simulink model "PubIfChassisHMI_MDL_DS"  (R2020b)
settings: configuration reference "DspaceConfig" (kept outside this file)
PostLoadFcn:
  | if any(exist('dsrtsu_mdlpostloadfcn', 'file') ~= 0), dsrtsu_mdlpostloadfcn('Execute', bdroot); end
InitFcn:
  | , if any(exist('rtifpga_mdlclblib', 'file') ~= 0), rtifpga_mdlclblib('Init', bdroot); end,
  | , if any(exist('dsmpb_private', 'file') ~= 0), dsmpb_private('dsmpb_mdlclblib', 'Init', bdroot); end,
PreSaveFcn:
  | , if any(exist('dsmpb_private', 'file') ~= 0), dsmpb_private('dsmpb_mdlclblib', 'PreSave', bdroot); end,
CloseFcn:
  | , if any(exist('dsmpb_private', 'file') ~= 0), dsmpb_private('dsmpb_mdlclblib', 'Close', bdroot); end,
settings Model: DataDictionary=HMI_Parameter.sldd  RTICANMMDATA=struct('GeneralSetupData',struct('modelroot','E:\HWA_Project\Git_ADAS_Store\projcct\adas_project\AdasModel_DSconfig','generalsettings',struct('filesettings',struct('destfolder',struct('Name','RTICANMM_FILES','Check',1),'buildfolder',struct('Name','.','Check',1),'AbsDestfolder',struct('Name','E:\HWA_Project\Git_ADAS_Store\projcct\adas_project\AdasModel_DSconfig\RTICANMM_FILES'),'AbsBuildfolder',struct('Name','E:\HWA_Project\Git_ADAS_Store\projcct\adas_project\AdasModel_DSconfig'))),'options',struct('addpaths',1,'rmpaths',1,'addtrcexclusion',false,'cannavigator',struct('checkmonitoring',0),'show_usrtrc',0,'use_usrtrc',0),'advanced',struct('options',ones(1,100)),'MPSetup',{{}},'RTI',struct('Type','DSRT','Ver','4.4','Date','02-Nov-2020'),'modelname','PubIfChassisHMI_MDL_DS','block','PubIfChassisHMI_MDL_DS'))  DSRTSU_INTERNAL_RTIFPGA=170  Creator=GW00180895  LastModifiedBy=GW00201299
settings ConfigSetRef: SourceName=DspaceConfig

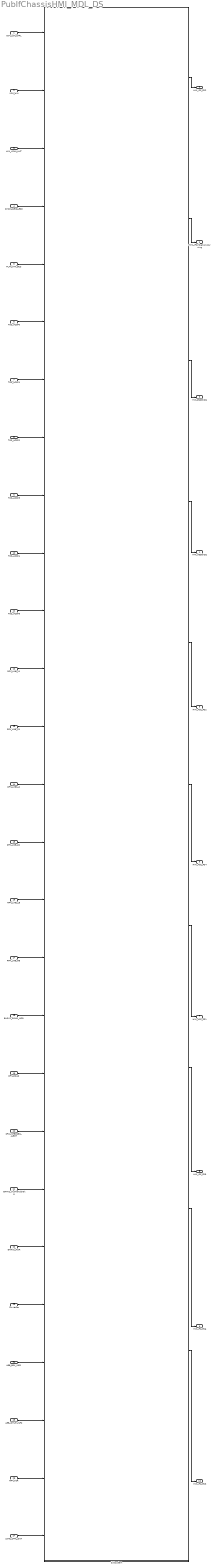
== system PubIfChassisHMI_MDL_DS ==
  VSM_LON_CTRL : Inport  OutDataTypeStr=Bus: VSM_LON_CTRL_BUS  PortDimensions=1  BusOutputAsStruct=on
  VSM_HMI : Inport  Port=2  OutDataTypeStr=Bus: VSM_HMI_BUS  PortDimensions=1  BusOutputAsStruct=on
  HMI_VCAN_HUT : Inport  Port=3  OutDataTypeStr=Bus: VCAN_HUT_MSG_BUS  PortDimensions=1  BusOutputAsStruct=on
  DMON_SENS_ERR : Inport  Port=4  OutDataTypeStr=Bus: DMON_SENS_ERR_BUS  PortDimensions=1  BusOutputAsStruct=on
  PLAN_HMI_BUS : Inport  Port=5  OutDataTypeStr=Bus: PLAN_HMI_BUS  PortDimensions=1  BusOutputAsStruct=on
  TOS_ACCP0 : Inport  Port=6  OutDataTypeStr=Bus: TOS_ACCP0_BUS  PortDimensions=1  BusOutputAsStruct=on
  TOS_ACCP1 : Inport  Port=7  OutDataTypeStr=Bus: TOS_ACCP1_BUS  PortDimensions=1  BusOutputAsStruct=on
  TOS_ACCP2 : Inport  Port=8  OutDataTypeStr=Bus: TOS_ACCP2_BUS  PortDimensions=1  BusOutputAsStruct=on
  TOS_ACCP3 : Inport  Port=9  OutDataTypeStr=Bus: TOS_ACCP3_BUS  PortDimensions=1  BusOutputAsStruct=on
  TOS_ACCP4 : Inport  Port=10  OutDataTypeStr=Bus: TOS_ACCP4_BUS  PortDimensions=1  BusOutputAsStruct=on
  TOS_ACCP5 : Inport  Port=11  OutDataTypeStr=Bus: TOS_ACCP5_BUS  PortDimensions=1  BusOutputAsStruct=on
  RFM_LINE_L1 : Inport  Port=12  OutDataTypeStr=Bus: RFM_LINE_BUS  PortDimensions=1  BusOutputAsStruct=on
  RFM_LINE_R1 : Inport  Port=13  OutDataTypeStr=Bus: RFM_LINE_BUS  PortDimensions=1  BusOutputAsStruct=on
  RFM_LINE_L2 : Inport  Port=14  OutDataTypeStr=Bus: RFM_LINE_BUS  PortDimensions=1  BusOutputAsStruct=on
  RFM_LINE_R2 : Inport  Port=15  OutDataTypeStr=Bus: RFM_LINE_BUS  PortDimensions=1  BusOutputAsStruct=on
  RFM_LINE_LB : Inport  Port=16  OutDataTypeStr=Bus: RFM_LINE_BUS  PortDimensions=1  BusOutputAsStruct=on
  RFM_LINE_RB : Inport  Port=17  OutDataTypeStr=Bus: RFM_LINE_BUS  PortDimensions=1  BusOutputAsStruct=on
  EHRV2_ROAD_INFO : Inport  Port=18  OutDataTypeStr=Bus: EHRV2_ROAD_INFO_BUS  PortDimensions=1  BusOutputAsStruct=on
  RFM_ROAD : Inport  Port=19  OutDataTypeStr=Bus: RFM_ROAD_BUS  PortDimensions=1  BusOutputAsStruct=on
  RFM_INTERSEC_ALERT : Inport  Port=20  OutDataTypeStr=Bus: RFM_INTERSEC_ALERT_BUS  PortDimensions=1  BusOutputAsStruct=on
  EHRV2_HutHandshake : Inport  Port=21  OutDataTypeStr=uint8  PortDimensions=1  BusOutputAsStruct=on
  EHRV2_HDR : Inport  Port=22  OutDataTypeStr=Bus: EHRV2_HDR_BUS  PortDimensions=1  BusOutputAsStruct=on
  DriverSts : Inport  Port=23  OutDataTypeStr=uint8  PortDimensions=1  BusOutputAsStruct=on
  AEB_BRK_INFO : Inport  Port=24  OutDataTypeStr=Bus: AEB_BRK_INFO_BUS  PortDimensions=1  BusOutputAsStruct=on
  AEB_IPHUT_INFO : Inport  Port=25  OutDataTypeStr=Bus: AEB_IPHUT_INFO_BUS  PortDimensions=1  BusOutputAsStruct=on
  RFM_TSR : Inport  Port=26  OutDataTypeStr=Bus: RFM_TSR_BUS  PortDimensions=1  BusOutputAsStruct=on
  LONC_CTRL_OUT : Inport  Port=27  OutDataTypeStr=Bus: LONC_CTRL_OUT_BUS  PortDimensions=1  BusOutputAsStruct=on
  Subsystem : Subsystem  ReferencedSubsystem=PvtSubSys_HMI
  HMI_IFC_FD2 : Outport  OutDataTypeStr=Bus: HMI_IFC_FD2_BUS  PortDimensions=1  BusOutputAsStruct=on
  HMI_IFCVibrationWarning : Outport  Port=2  OutDataTypeStr=uint8  PortDimensions=1  BusOutputAsStruct=on
  HMI_ESSErrSts : Outport  Port=3  OutDataTypeStr=boolean  BusOutputAsStruct=on
  HMI_AESErrSts : Outport  Port=4  OutDataTypeStr=boolean  BusOutputAsStruct=on
  HMI_ACC_FD2 : Outport  Port=5  OutDataTypeStr=Bus: HMI_ACC_FD2_BUS  PortDimensions=1  BusOutputAsStruct=on
  HMI_ACC_FD4 : Outport  Port=6  OutDataTypeStr=Bus: HMI_ACC_FD4_BUS  PortDimensions=1  BusOutputAsStruct=on
  HMI_ACC_FD1 : Outport  Port=7  OutDataTypeStr=Bus: HMI_ACC_FD1_BUS  PortDimensions=1  BusOutputAsStruct=on
  HMI_IFC_FD5 : Outport  Port=8  OutDataTypeStr=Bus: HMI_IFC_FD5_BUS  PortDimensions=1  BusOutputAsStruct=on
  HMI_IFC_FD6 : Outport  Port=9  OutDataTypeStr=Bus: HMI_IFC_FD6_BUS  PortDimensions=1  BusOutputAsStruct=on
  HMI_IFC_FD3 : Outport  Port=10  OutDataTypeStr=Bus: HMI_IFC_FD3_BUS  PortDimensions=1  BusOutputAsStruct=on
  wires:
  RFM_LINE_L1/1 -> Subsystem/12
  Subsystem/10 -> HMI_IFC_FD3/1
  Subsystem/2 -> HMI_IFCVibrationWarning/1
  Subsystem/4 -> HMI_AESErrSts/1
  AEB_IPHUT_INFO/1 -> Subsystem/25
  Subsystem/5 -> HMI_ACC_FD2/1
  TOS_ACCP0/1 -> Subsystem/6
  Subsystem/9 -> HMI_IFC_FD6/1
  TOS_ACCP2/1 -> Subsystem/8
  Subsystem/7 -> HMI_ACC_FD1/1
  Subsystem/3 -> HMI_ESSErrSts/1
  Subsystem/6 -> HMI_ACC_FD4/1
  Subsystem/8 -> HMI_IFC_FD5/1
  VSM_HMI/1 -> Subsystem/2
  RFM_INTERSEC_ALERT/1 -> Subsystem/20
  Subsystem/1 -> HMI_IFC_FD2/1
  TOS_ACCP4/1 -> Subsystem/10
  LONC_CTRL_OUT/1 -> Subsystem/27
  RFM_TSR/1 -> Subsystem/26
  AEB_BRK_INFO/1 -> Subsystem/24
  DriverSts/1 -> Subsystem/23
  RFM_LINE_L2/1 -> Subsystem/14
  EHRV2_HDR/1 -> Subsystem/22
  EHRV2_HutHandshake/1 -> Subsystem/21
  RFM_ROAD/1 -> Subsystem/19
  HMI_VCAN_HUT/1 -> Subsystem/3
  EHRV2_ROAD_INFO/1 -> Subsystem/18
  RFM_LINE_RB/1 -> Subsystem/17
  RFM_LINE_LB/1 -> Subsystem/16
  RFM_LINE_R2/1 -> Subsystem/15
  RFM_LINE_R1/1 -> Subsystem/13
  TOS_ACCP5/1 -> Subsystem/11
  TOS_ACCP3/1 -> Subsystem/9
  TOS_ACCP1/1 -> Subsystem/7
  PLAN_HMI_BUS/1 -> Subsystem/5
  DMON_SENS_ERR/1 -> Subsystem/4
  VSM_LON_CTRL/1 -> Subsystem/1
